simulink model "MoboticStartup_TimingSync"  (R2024a)
settings: Solver=FixedStepAuto  StartTime=0.0  StopTime=inf  RelTol=1e-3
settings Model: DataDictionary=configuration_dictionary.sldd  Creator=matlab.cut  LastModifiedBy=matlab.cut
settings SolverCC: ConcurrentTasks=on  PositivePriorityOrder=on
settings OptimizationCC: BlockReduction=off  DefaultParameterBehavior=Inlined  OptimizeBlockIOStorage=off
settings DebuggingCC: UnderspecifiedInitializationDetection=Classic  TasksWithSamePriorityMsg=none
settings HardwareCC: ProdBitPerLong=64  ProdLongLongMode=on  ProdHWDeviceType=Intel->x86-64 (Linux 64)
settings ModelReferenceCC: ModelReferenceNumInstancesAllowed=Single
settings SFSimCC: MATLABDynamicMemAlloc=off
settings RTWCC: Description=Speedgoat Real-Time Target Machine  SystemTargetFile=speedgoat.tlc  TemplateMakefile=slrealtime_default_tmf  Toolchain=Simulink Real-Time Toolchain  BuildConfiguration=Faster Runs  CodeExecutionProfiling=on  TargetLang=C++
settings CodeAppCC: MaxIdLength=127
settings SimulinkRealTimeTargetCC: InstructionSetFMA=off  LogToMDFFile=off

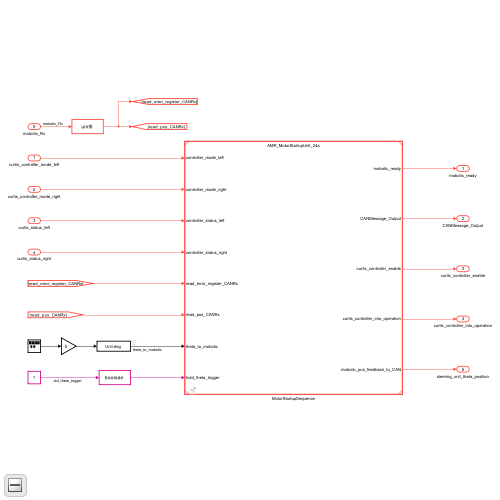
[thumbnail: Simulink's stored preview of the top-level diagram]
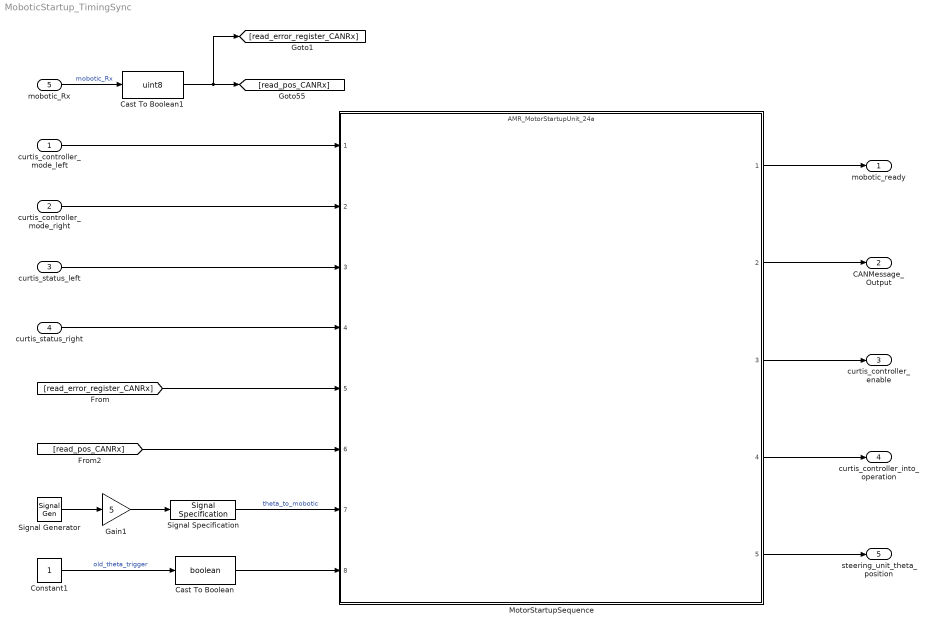
== system MoboticStartup_TimingSync ==
  curtis_controller_mode_left : Inport
  curtis_controller_mode_right : Inport  Port=2
  curtis_status_left : Inport  Port=3
  curtis_status_right : Inport  Port=4
  mobotic_Rx : Inport  Port=5
  Cast To Boolean : DataTypeConversion  OutDataTypeStr=boolean  SaturateOnIntegerOverflow=off  RndMeth=Floor
  Cast To Boolean1 : DataTypeConversion  OutDataTypeStr=uint8  SaturateOnIntegerOverflow=off  RndMeth=Floor
  Constant1 : Constant
  Gain1 : Gain  Gain=5
  MotorStartupSequence : ModelReference  ModelNameDialog=AMR_MotorStartupUnit_24a.slx  SimulationMode=Normal  ModelReferenceVersion=2.43
  Signal Generator : SignalGenerator  Frequency=0.1
  Signal Specification : SignalSpecification  Unit=deg
  mobotic_ready : Outport
  CANMessage_Output : Outport  Port=2
  curtis_controller_enable : Outport  Port=3
  curtis_controller_into_operation : Outport  Port=4
  steering_unit_theta_position : Outport  Port=5
  wires:
  curtis_controller_mode_left/1 -> MotorStartupSequence/1
  curtis_controller_mode_right/1 -> MotorStartupSequence/2
  curtis_status_right/1 -> MotorStartupSequence/4
  curtis_status_left/1 -> MotorStartupSequence/3
  MotorStartupSequence/1 -> mobotic_ready/1
  mobotic_Rx/1 -> Cast To Boolean1/1  "mobotic_Rx"
  MotorStartupSequence/2 -> CANMessage_Output/1
  MotorStartupSequence/4 -> curtis_controller_into_operation/1
  MotorStartupSequence/3 -> curtis_controller_enable/1
  Gain1/1 -> Signal Specification/1
  Constant1/1 -> Cast To Boolean/1  "old_theta_trigger"
  MotorStartupSequence/5 -> steering_unit_theta_position/1
  Signal Generator/1 -> Gain1/1
  Cast To Boolean/1 -> MotorStartupSequence/8
  Signal Specification/1 -> MotorStartupSequence/7  "theta_to_mobotic"
  [read_pos_CANRx] -> MotorStartupSequence/6
  [read_error_register_CANRx] -> MotorStartupSequence/5
  Cast To Boolean1/1 -> [read_pos_CANRx], [read_error_register_CANRx]
